simulink model "heli_q8"  (R2014a)
settings: Solver=ode1  StartTime=0.0  StopTime=inf  FixedStep=0.002  RelTol=1e-3
PostLoadFcn:
  | qc_set_target_type(getConfigSet(bdroot, 'QUARC Default Target Configuration'));
values from neighbouring files (symbols this model uses):
  A = [0 1 0 0 0 0; 0 0 0 0 0 0; 0 0 0 1 0 0; 0 0 0 0 0 0; 0 0 0 0 0 1; K_3 0 0 0 0 0]    [init_heli_all.m]
  B = [0 0; 0 K_1; 0 0; K_2 0; 0 0; 0 0]    [init_heli_all.m]
  C = [1 0 0 0 0 0; 0 0 1 0 0 0; 0 0 0 0 1 0]    [init_heli_all.m]
  Joystick_gain_x = 1    [init_heli_all.m]
  Joystick_gain_y = -1    [init_heli_all.m]
  K_v2 = lqr(A_v2,B_v2,Q_v2,R_v2)    [init_heli_all.m]
  L = place(A',C',poles)'    [init_heli_all.m]
  P_v1 = inv(C_v1*inv(-A_v1+B_v1*K_v1)*B_v1)    [init_heli_all.m]
undefined symbols (not defined in the file or in its folder): HIL, qc_get_step_size
libraries: simulink_extras x6, quarc_library x4
settings Model: SimulationMode=external  ExtModeTrigDuration=5000  Creator=Rchan  LastModifiedBy=magneasi
settings SolverCC: PositivePriorityOrder=on
settings DataIOCC: SignalLoggingSaveFormat=ModelDataLogs
settings OptimizationCC: ExpressionDepthLimit=2147483647  InitFltsAndDblsToZero=on
settings DebuggingCC: SaveWithParameterizedLinksMsg=none  UnderspecifiedInitializationDetection=Classic  MultiTaskDSMMsg=warning  MultiTaskCondExecSysMsg=none  FcnCallInpInsideContextMsg=UseLocalSettings  StateNameClashWarn=warning
settings RTWCC: SystemTargetFile=quarc_win64.tlc  TemplateMakefile=quarc_default_tmf  Description=QUARC Win64 Target  ProcessScript=quarc_win64_make_rtw_hook
settings STFCustomTargetCC: CPPClassGenCompliant=on
settings GRTTargetCC: ParMdlRefBuildCompliant=off  CompOptLevelCompliant=off  CombineOutputUpdateFcns=off  MatFileLogging=off  GRTInterface=on  ExtMode=on  ExtModeMexFile=quarc_comm

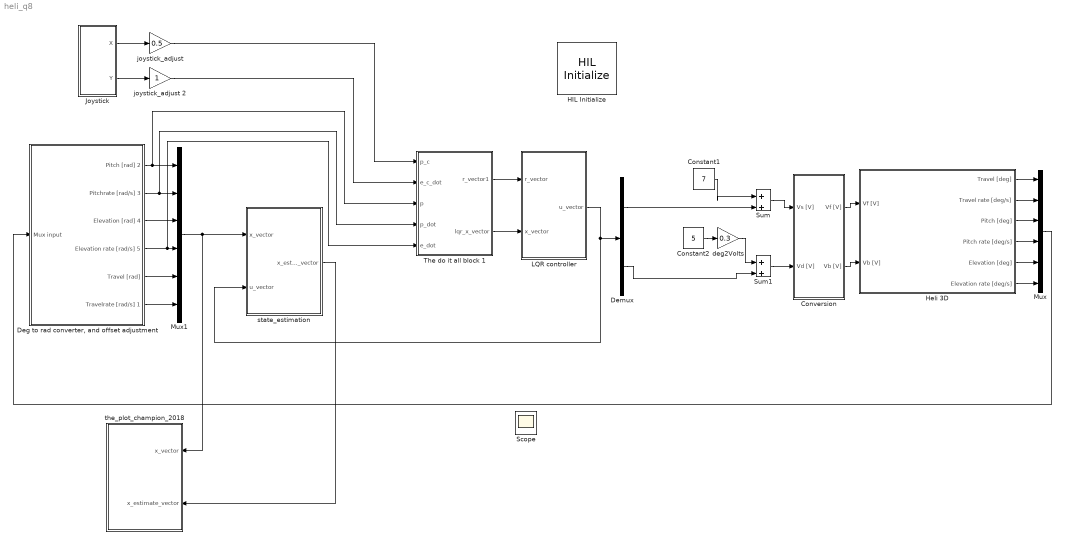
== system heli_q8 ==
  Constant1 : Constant  Value=7
  Constant2 : Constant  Value=5
  Conversion : Subsystem
  "Deg to rad converter, and offset adjustment " : Subsystem
  Demux : Demux  Outputs=2
  HIL Initialize : quarc_library/Data Acquisition/Generic/Configuration/HIL Initialize  Priority=-99  object_name=HIL-1  board_type=q8_usb  board_number=0  board_options=update_rate=normal;decimation=1  exclusive=off  active=off  hardware_clocks=[0:2]  clock_modes=[]  initial_clock_frequencies=[]  set_clock_params_at_start=off  set_clock_params_at_switch_in=off  set_clock_frequencies_at_start=off  set_clock_frequencies_at_switch_in=off  analog_input_channels=[0:7]  analog_input_maximums=10  analog_input_minimums=-10  set_analog_input_params_at_start=on  set_analog_input_params_at_switch_in=off  analog_output_channels=[0:7]  analog_output_maximums=10  analog_output_minimums=-10  initial_analog_outputs=[0]  final_analog_outputs=[0]  watchdog_analog_outputs=0  set_analog_output_params_at_start=on  set_analog_output_params_at_switch_in=off  set_analog_outputs_at_start=on  set_analog_outputs_at_switch_in=off  set_analog_outputs_at_terminate=on  set_analog_outputs_at_switch_out=off  set_analog_outputs_on_watchdog=off  digital_input_channels=[]  digital_output_channels=[]  digital_output_configuration=[]  initial_digital_outputs=[1]  final_digital_outputs=[1]  watchdog_digital_outputs=[1]  set_digital_output_params_at_start=off  set_digital_output_params_at_switch_in=off  set_digital_outputs_at_start=on  set_digital_outputs_at_switch_in=off  set_digital_outputs_at_terminate=on  set_digital_outputs_at_switch_out=off  set_digital_outputs_on_watchdog=off  encoder_channels=[0:7]  quadrature=[4]  encoder_filter_frequency=[]  initial_encoder_counts=[0]  set_encoder_params_at_start=on  set_encoder_params_at_switch_in=off  set_encoder_counts_at_start=on  set_encoder_counts_at_switch_in=off  pwm_channels=[0:7]  pwm_modes=0  pwm_frequency=99.532799999999995e6/4095  pwm_configuration=[0]  pwm_alignment=[0]  pwm_polarity=[1]  pwm_leading_deadband=[0]  pwm_trailing_deadband=[0]  initial_pwm_outputs=[0]  final_pwm_outputs=[0]  watchdog_pwm_outputs=[0]  set_pwm_params_at_start=on  set_pwm_params_at_switch_in=off  set_pwm_outputs_at_start=on  set_pwm_outputs_at_switch_in=off  set_pwm_outputs_at_terminate=on  set_pwm_outputs_at_switch_out=off  set_pwm_outputs_on_watchdog=off  other_output_channels=[]  initial_other_outputs=[]  final_other_outputs=[]  watchdog_other_outputs=[]  set_other_outputs_at_start=off  set_other_outputs_at_switch_in=off  set_other_outputs_at_terminate=off  set_other_outputs_at_switch_out=off  set_other_outputs_on_watchdog=off
  Heli 3D : Subsystem
  Joystick : Subsystem
  LQR controller : Subsystem
  Mux : Mux  Inputs=6
  Mux1 : Mux  Inputs=6
  Scope : Scope
      settings: ShowLegends=on  YMin=-3  YMax=17
  Sum : Sum  Inputs=|++
  Sum1 : Sum  Inputs=|++
  The do it all block 1 : Subsystem
  deg2Volts : Gain  Gain=0.3
  "joystick_adjust " : Gain  Gain=0.5
  joystick_adjust 2 : Gain
  state_estimation : Subsystem
  the_plot_champion_2018 : Subsystem
  wires:
  Conversion/2(Vb [V]) -> Heli 3D/2(Vb [V])
  Conversion/1(Vf [V]) -> Heli 3D/1(Vf [V])
  Heli 3D/1(Travel [deg]) -> Mux/1
  Heli 3D/2(Travel rate [deg/s]) -> Mux/2
  Heli 3D/3(Pitch [deg]) -> Mux/3
  Heli 3D/4(Pitch rate [deg/s]) -> Mux/4
  Heli 3D/5(Elevation [deg]) -> Mux/5
  Heli 3D/6(Elevation rate [deg/s]) -> Mux/6
  Mux/1 -> "Deg to rad converter, and offset adjustment "/1("Mux input ")
  Joystick/1(X) -> "joystick_adjust "/1
  "joystick_adjust "/1 -> The do it all block 1/1(p_c)
  joystick_adjust 2/1 -> The do it all block 1/2("e_c_dot ")
  Joystick/2(Y) -> joystick_adjust 2/1
  Demux/1 -> Sum/2
  Sum/1 -> Conversion/1(Vs [V])
  Constant1/1 -> Sum/1
  Demux/2 -> Sum1/2
  Sum1/1 -> Conversion/2(Vd [V])
  Constant2/1 -> deg2Volts/1
  deg2Volts/1 -> Sum1/1
  "Deg to rad converter, and offset adjustment "/1(Pitch [rad] 2) -> Mux1/1, The do it all block 1/3("p ")
  "Deg to rad converter, and offset adjustment "/2(Pitchrate [rad/s] 3) -> Mux1/2, The do it all block 1/4(p_dot)
  "Deg to rad converter, and offset adjustment "/3(Elevation [rad] 4) -> Mux1/3
  "Deg to rad converter, and offset adjustment "/4(Elevation rate [rad/s] 5) -> The do it all block 1/5(e_dot), Mux1/4
  "Deg to rad converter, and offset adjustment "/5("Travel [rad] ") -> Mux1/5
  "Deg to rad converter, and offset adjustment "/6(Travelrate [rad/s] 1) -> Mux1/6
  The do it all block 1/2(lqr_x_vector) -> LQR controller/2(x_vector)
  The do it all block 1/1(r_vector1) -> LQR controller/1(r_vector)
  LQR controller/1(u_vector) -> Demux/1, state_estimation/2(u_vector)
  Mux1/1 -> the_plot_champion_2018/1("x_vector "), state_estimation/1("x_vector ")
  state_estimation/1(x_estimation_vector) -> the_plot_champion_2018/2(x_estimate_vector)

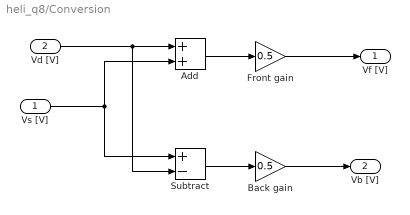
== system heli_q8/Conversion ==
  Vs [V] : Inport
  Vd [V] : Inport  Port=2
  Add : Sum
  Back gain : Gain  Gain=0.5
  Front gain : Gain  Gain=0.5
  Subtract : Sum  Inputs=+-
  Vf [V] : Outport
  Vb [V] : Outport  Port=2
  wires:
  Vd [V]/1 -> Subtract/2, Add/1
  Vs [V]/1 -> Subtract/1, Add/2
  Subtract/1 -> Back gain/1
  Back gain/1 -> Vb [V]/1
  Add/1 -> Front gain/1
  Front gain/1 -> Vf [V]/1

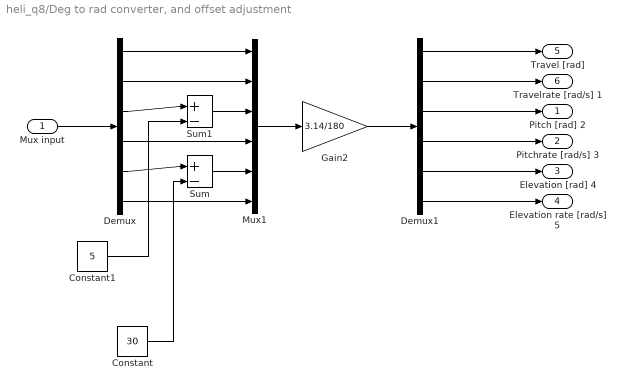
== system heli_q8/Deg to rad converter, and offset adjustment  ==
  "Mux input " : Inport
  Constant : Constant  Value=30
  Constant1 : Constant  Value=5
  Demux : Demux  Outputs=6
  Demux1 : Demux  Outputs=6
  Gain2 : Gain  Gain=3.14/180
  Mux1 : Mux  Inputs=6
  Sum : Sum  Inputs=|+-
  Sum1 : Sum  Inputs=|+-
  Pitch [rad] 2 : Outport
  Pitchrate [rad/s] 3 : Outport  Port=2
  Elevation [rad] 4 : Outport  Port=3
  Elevation rate [rad/s] 5 : Outport  Port=4
  "Travel [rad] " : Outport  Port=5
  Travelrate [rad/s] 1 : Outport  Port=6
  wires:
  "Mux input "/1 -> Demux/1
  Demux/5 -> Sum/1
  Demux1/5 -> Elevation [rad] 4/1
  Constant/1 -> Sum/2
  Gain2/1 -> Demux1/1
  Demux1/3 -> Pitch [rad] 2/1
  Demux1/4 -> Pitchrate [rad/s] 3/1
  Demux1/6 -> Elevation rate [rad/s] 5/1
  Demux/1 -> Mux1/1
  Demux/6 -> Mux1/6
  Demux/4 -> Mux1/4
  Demux1/1 -> "Travel [rad] "/1
  Mux1/1 -> Gain2/1
  Sum/1 -> Mux1/5
  Demux1/2 -> Travelrate [rad/s] 1/1
  Demux/2 -> Mux1/2
  Demux/3 -> Sum1/1
  Sum1/1 -> Mux1/3
  Constant1/1 -> Sum1/2

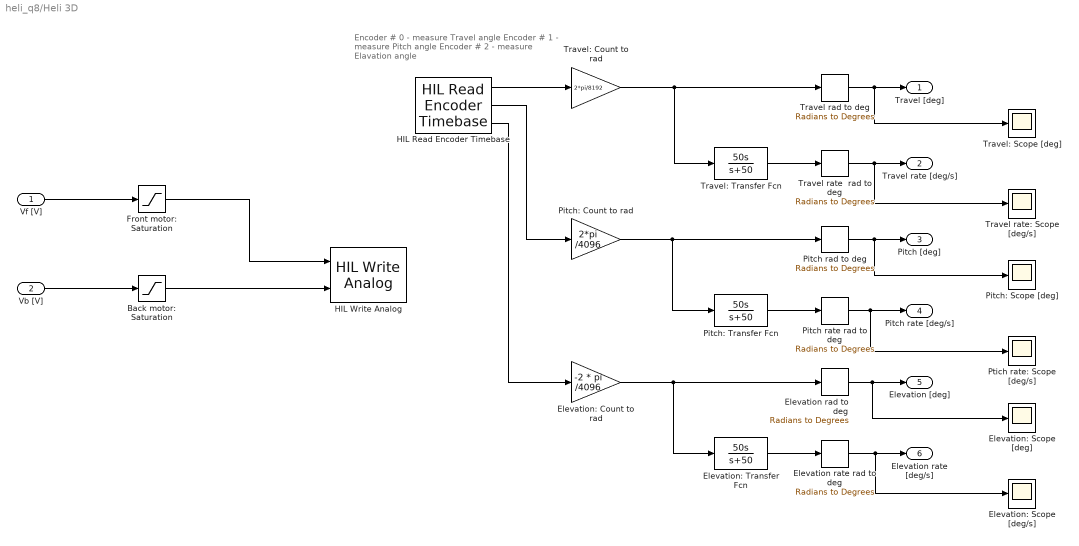
== system heli_q8/Heli 3D ==
  note: Encoder # 0 - measure Travel angle
      | Encoder # 1 - measure Pitch angle
      | Encoder # 2 - measure Elavation angle
  Vf [V] : Inport
  Vb [V] : Inport  Port=2
  Back motor: Saturation : Saturate  UpperLimit=5  LowerLimit=-5
  Elevation rad to deg : simulink_extras/Transformations/Radians to Degrees
  Elevation rate rad to deg : simulink_extras/Transformations/Radians to Degrees
  Elevation: Count to rad : Gain  Gain=-2 * pi /4096
  Elevation: Scope [deg/s] : Scope
      settings: YMin=-15  YMax=15  SaveName=ScopeData13
  Elevation: Scope [deg] : Scope
      settings: YMin=-0  YMax=32.5  SaveName=ScopeData12
  Elevation: Transfer Fcn : TransferFcn  Numerator=[50 0]  Denominator=[1 50]
  Front motor: Saturation : Saturate  UpperLimit=5  LowerLimit=-5
  HIL Read Encoder Timebase : quarc_library/Data Acquisition/Generic/Timebases/HIL Read Encoder Timebase  object_name=HIL-1  clock=0  channels=[0:2]  samples_in_buffer=max(ceil(1/qc_get_step_size), 1)  active=on  vector_output=off  data_type_mode=Inherit via back propagation  data_type=double
  HIL Write Analog : quarc_library/Data Acquisition/Generic/Immediate I//O/HIL Write Analog  object_name=HIL-1  channels=[0:1]  sample_time=-1  active=off  vector_input=off
  Pitch rad to deg : simulink_extras/Transformations/Radians to Degrees
  Pitch rate rad to deg : simulink_extras/Transformations/Radians to Degrees
  Pitch: Count to rad : Gain  Gain=2*pi /4096
  Pitch: Scope [deg] : Scope
      settings: YMin=-45  YMax=2.5  SaveName=ScopeData10
  Pitch: Transfer Fcn : TransferFcn  Numerator=[50 0]  Denominator=[1 50]
  Ptich rate: Scope [deg/s] : Scope
      settings: YMin=-15  YMax=15  SaveName=ScopeData11
  Travel rad to deg : simulink_extras/Transformations/Radians to Degrees
  Travel rate  rad to deg : simulink_extras/Transformations/Radians to Degrees
  Travel rate: Scope [deg/s] : Scope
      settings: YMin=-15  YMax=15  SaveName=ScopeData9
  Travel: Count to rad : Gain  Gain=2*pi/8192
  Travel: Scope [deg] : Scope
      settings: YMin=-45  YMax=12.5  SaveName=ScopeData8
  Travel: Transfer Fcn : TransferFcn  Numerator=[50 0]  Denominator=[1 50]
  Travel [deg] : Outport
  Travel rate [deg/s] : Outport  Port=2
  Pitch [deg] : Outport  Port=3
  Pitch rate [deg/s] : Outport  Port=4
  Elevation [deg] : Outport  Port=5
  Elevation rate [deg/s] : Outport  Port=6
  wires:
  HIL Read Encoder Timebase/1 -> Travel: Count to rad/1
  HIL Read Encoder Timebase/2 -> Pitch: Count to rad/1
  HIL Read Encoder Timebase/3 -> Elevation: Count to rad/1
  Travel: Count to rad/1 -> Travel: Transfer Fcn/1, Travel rad to deg/1
  Travel: Transfer Fcn/1 -> Travel rate  rad to deg/1
  Pitch: Count to rad/1 -> Pitch: Transfer Fcn/1, Pitch rad to deg/1
  Pitch: Transfer Fcn/1 -> Pitch rate rad to deg/1
  Elevation: Count to rad/1 -> Elevation: Transfer Fcn/1, Elevation rad to deg/1
  Elevation: Transfer Fcn/1 -> Elevation rate rad to deg/1
  Travel rad to deg/1 -> Travel: Scope [deg]/1, Travel [deg]/1
  Travel rate  rad to deg/1 -> Travel rate: Scope [deg/s]/1, Travel rate [deg/s]/1
  Pitch rad to deg/1 -> Pitch: Scope [deg]/1, Pitch [deg]/1
  Pitch rate rad to deg/1 -> Ptich rate: Scope [deg/s]/1, Pitch rate [deg/s]/1
  Elevation rad to deg/1 -> Elevation: Scope [deg]/1, Elevation [deg]/1
  Elevation rate rad to deg/1 -> Elevation: Scope [deg/s]/1, Elevation rate [deg/s]/1
  Vf [V]/1 -> Front motor: Saturation/1
  Vb [V]/1 -> Back motor: Saturation/1
  Front motor: Saturation/1 -> HIL Write Analog/1
  Back motor: Saturation/1 -> HIL Write Analog/2

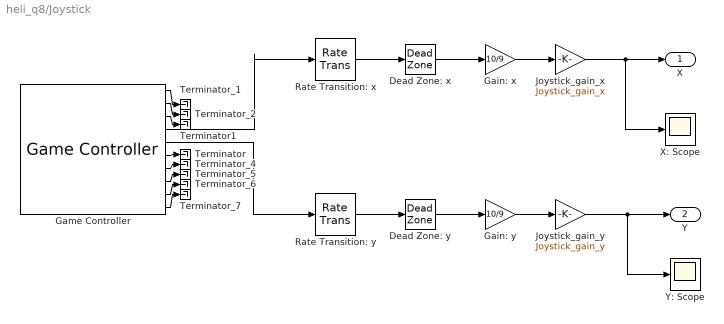
== system heli_q8/Joystick ==
  Dead Zone: x : DeadZone  LowerValue=-0.1  UpperValue=0.1  SaturateOnIntegerOverflow=on
  Dead Zone: y : DeadZone  LowerValue=-0.1  UpperValue=0.1  SaturateOnIntegerOverflow=on
  Gain: x : Gain  Gain=10/9
  Gain: y : Gain  Gain=10/9
  Game Controller : quarc_library/Devices/Peripherals/Target/Game Controller  controller=1  buffer_size=12  deadzone=[]  saturation=[]  sample_time=max(qc_get_step_size, 0.01)  auto_center=off  enabled=on
  Joystick_gain_x : Gain  Gain=Joystick_gain_x
  Joystick_gain_y : Gain  Gain=Joystick_gain_y
  Rate Transition: x : RateTransition
  Rate Transition: y : RateTransition
  Terminator : Terminator
  Terminator1 : Terminator
  Terminator_{1..2,4..7} (6 alike) : Terminator
  X: Scope : Scope
      settings: YMin=-1  YMax=1  SaveName=ScopeData7
  Y: Scope : Scope
      settings: YMin=-10  YMax=10  SaveName=ScopeData5
  X : Outport
  Y : Outport  Port=2
  wires:
  Rate Transition: y/1 -> Dead Zone: y/1
  Rate Transition: x/1 -> Dead Zone: x/1
  Game Controller/5 -> Rate Transition: y/1
  Game Controller/4 -> Rate Transition: x/1
  Game Controller/1 -> Terminator_1/1
  Game Controller/2 -> Terminator_2/1
  Game Controller/7 -> Terminator_4/1
  Game Controller/8 -> Terminator_5/1
  Game Controller/9 -> Terminator_6/1
  Game Controller/10 -> Terminator_7/1
  Game Controller/3 -> Terminator1/1
  Game Controller/6 -> Terminator/1
  Dead Zone: x/1 -> Gain: x/1
  Dead Zone: y/1 -> Gain: y/1
  Gain: x/1 -> Joystick_gain_x/1
  Gain: y/1 -> Joystick_gain_y/1
  Joystick_gain_x/1 -> X/1, X: Scope/1
  Joystick_gain_y/1 -> Y: Scope/1, Y/1

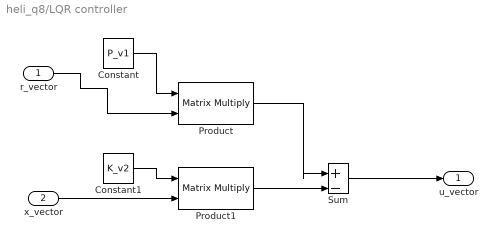
== system heli_q8/LQR controller ==
  r_vector : Inport
  x_vector : Inport  Port=2
  Constant : Constant  Value=P_v1
  Constant1 : Constant  Value=K_v2
  Product : Product  Multiplication=Matrix(*)
  Product1 : Product  Multiplication=Matrix(*)
  Sum : Sum  Inputs=|+-
  u_vector : Outport
  wires:
  Constant1/1 -> Product1/1
  r_vector/1 -> Product/2
  Product1/1 -> Sum/2
  x_vector/1 -> Product1/2
  Product/1 -> Sum/1
  Sum/1 -> u_vector/1
  Constant/1 -> Product/1

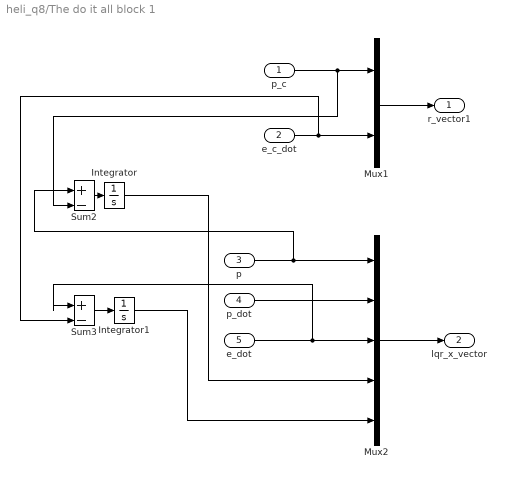
== system heli_q8/The do it all block 1 ==
  p_c : Inport
  "e_c_dot " : Inport  Port=2
  "p " : Inport  Port=3
  p_dot : Inport  Port=4
  e_dot : Inport  Port=5
  Integrator : Integrator
  Integrator1 : Integrator
  Mux1 : Mux  Inputs=2
  Mux2 : Mux  Inputs=5
  Sum2 : Sum  Inputs=|+-
  Sum3 : Sum  Inputs=|+-
  r_vector1 : Outport
  lqr_x_vector : Outport  Port=2
  wires:
  Mux2/1 -> lqr_x_vector/1
  p_dot/1 -> Mux2/2
  e_dot/1 -> Sum3/1, Mux2/3
  Integrator/1 -> Mux2/4
  Integrator1/1 -> Mux2/5
  "p "/1 -> Sum2/1, Mux2/1
  Mux1/1 -> r_vector1/1
  "e_c_dot "/1 -> Sum3/2, Mux1/2
  Sum3/1 -> Integrator1/1
  Sum2/1 -> Integrator/1
  p_c/1 -> Sum2/2, Mux1/1

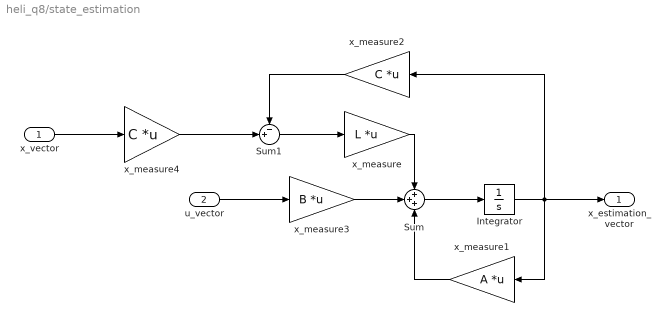
== system heli_q8/state_estimation ==
  "x_vector " : Inport
  u_vector : Inport  Port=2
  Integrator : Integrator
  Sum : Sum  Inputs=+++
  Sum1 : Sum  Inputs=-+|
  x_measure : Gain  Gain=L  Multiplication=Matrix(K*u)
  x_measure1 : Gain  Gain=A  Multiplication=Matrix(K*u)
  x_measure2 : Gain  Gain=C  Multiplication=Matrix(K*u)
  x_measure3 : Gain  Gain=B  Multiplication=Matrix(K*u)
  x_measure4 : Gain  Gain=C  Multiplication=Matrix(K*u)
  x_estimation_vector : Outport
  wires:
  u_vector/1 -> x_measure3/1
  Sum/1 -> Integrator/1
  Integrator/1 -> x_measure2/1, x_estimation_vector/1, x_measure1/1
  x_measure1/1 -> Sum/3
  x_measure/1 -> Sum/1
  x_measure2/1 -> Sum1/1
  Sum1/1 -> x_measure/1
  x_measure3/1 -> Sum/2
  "x_vector "/1 -> x_measure4/1
  x_measure4/1 -> Sum1/2

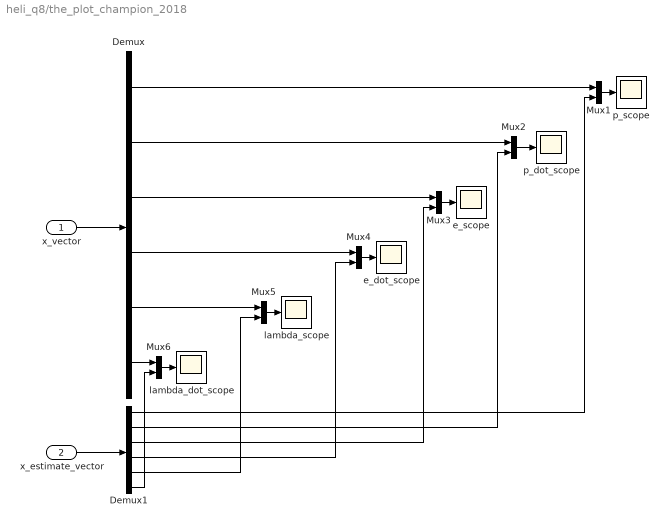
== system heli_q8/the_plot_champion_2018 ==
  "x_vector " : Inport
  x_estimate_vector : Inport  Port=2
  Demux : Demux  Outputs=6
  Demux1 : Demux  Outputs=6
  Mux{1..6} (6 alike) : Mux  Inputs=2
  e_dot_scope : Scope
      settings: ShowLegends=on  SaveName=ScopeData4
  e_scope : Scope
      settings: ShowLegends=on  SaveName=ScopeData3
  lambda_dot_scope : Scope
      settings: ShowLegends=on  SaveName=ScopeData14
  lambda_scope : Scope
      settings: ShowLegends=on  SaveName=ScopeData6
  p_dot_scope : Scope
      settings: ShowLegends=on  SaveName=ScopeData2
  p_scope : Scope
      settings: ShowLegends=on
  wires:
  x_estimate_vector/1 -> Demux1/1
  "x_vector "/1 -> Demux/1
  Demux/1 -> Mux1/1
  Demux1/1 -> Mux1/2
  Demux/2 -> Mux2/1
  Demux1/2 -> Mux2/2
  Demux/3 -> Mux3/1
  Demux1/3 -> Mux3/2
  Demux/4 -> Mux4/1
  Demux1/4 -> Mux4/2
  Demux/5 -> Mux5/1
  Demux1/5 -> Mux5/2
  Demux/6 -> Mux6/1
  Demux1/6 -> Mux6/2
  Mux1/1 -> p_scope/1
  Mux2/1 -> p_dot_scope/1
  Mux3/1 -> e_scope/1
  Mux4/1 -> e_dot_scope/1
  Mux5/1 -> lambda_scope/1
  Mux6/1 -> lambda_dot_scope/1
